simulink model "ddc_model"  (R2023b)
settings: Solver=VariableStepDiscrete  StartTime=0.0  StopTime=DDC_LINEUP_param.endTime  RelTol=1e-3  EnableMultiTasking=on
PreLoadFcn:
  | % Run the setup script when the model is opened
  | setup_ddc_model;
InitFcn:
  | % Run the setup script again just before the
  | % model is run, so that any updates made
  | % after opening are applied.
  | 
  | setup_ddc_model;
StopFcn:
  | ddc_output_analysis;
values from neighbouring files (symbols this model uses):
  DDC_CM_multiplication_factor = 1    [setup_ddc_model.m]
  DDC_CM_NCO1_phase = [0 0 0 0]*2^DDC_LINEUP_param.Complex_NCO1.accum_bit_width    [setup_ddc_model.m]
  DDC_CM_NCO_sync = [0 0 0 0]    [setup_ddc_model.m]
  DDC_CM_number_of_bits_to_shift_left = 0    [setup_ddc_model.m]
undefined symbols (not defined in the file or in its folder): AdvDSPBChannelOutDisplay, COMPLEX_MIXER, DDC_LINEUP_param, dpoly, dspba_ChannelInVis, dspba_ChannelOutVis, dspba_internal_get_channel_ports, evalAionMaskParam, latency, lddc, lddc_lib, mixer_lib, primtype, value
libraries: DSPBAPrim x43, DSPBABase x15, simulink x10, DSPBAFilters x6, DSPBAModelBus x3, DSPBAWaveformSynth x2
(part 1 of 2)
Description:
  | DSP Builder Advanced Template for Template Design implementing ModelIP designs
settings Model: Creator=mjervis  LastModifiedBy=5g
settings SolverCC: AlgebraicLoopSolver=TrustRegion
settings DataIOCC: LimitDataPoints=on  SaveFormat=Array  SignalLoggingSaveFormat=ModelDataLogs  ReturnWorkspaceOutputs=off
settings OptimizationCC: ExpressionDepthLimit=2147483647  LifeSpan=inf
settings DebuggingCC: UnderspecifiedInitializationDetection=Classic  MergeDetectMultiDrivingBlocksExec=none  SolverPrmCheckMsg=warning  InheritedTsInSrcMsg=none  IntegerOverflowMsg=none  FcnCallInpInsideContextMsg=warning  UnconnectedInputMsg=warning  UnconnectedOutputMsg=warning  UnconnectedLineMsg=warning  StateNameClashWarn=warning  SFUnexpectedBacktrackingDiag=warning  SFNoUnconditionalDefaultTransitionDiag=warning  SFExecutionAtInitializationDiag=none  IntegerSaturationMsg=none  ArithmeticOperatorsInVariantConditions=warning
settings HardwareCC: ProdBitPerPointer=32  ProdBitPerSizeT=32  ProdBitPerPtrDiffT=32  ProdLargestAtomicFloat=None  ProdIntDivRoundTo=Undefined  ProdEndianess=Unspecified  ProdWordSize=32  ProdHWDeviceType=32-bit Generic
settings ModelReferenceCC: EnableRefExpFcnMdlSchedulingChecks=on  PropagateSignalLabelsOutOfModel=off
settings SFSimCC: SimUseLocalCustomCode=off  CustomCodeUndefinedFunction=UseInterfaceOnly
settings RTWCC: RTWUseLocalCustomCode=off  DLArmComputeVersion=19.05
settings CodeAppCC: StateflowObjectComments=on
settings GRTTargetCC: TargetLangStandard=C89/C90 (ANSI)  CombineOutputUpdateFcns=off  GRTInterface=on
settings ConfigComp: CovMetricSettings=dw  CovSaveCumulativeToWorkspaceVar=on  CovSaveSingleToWorkspaceVar=on  CovExternalEMLEnable=off

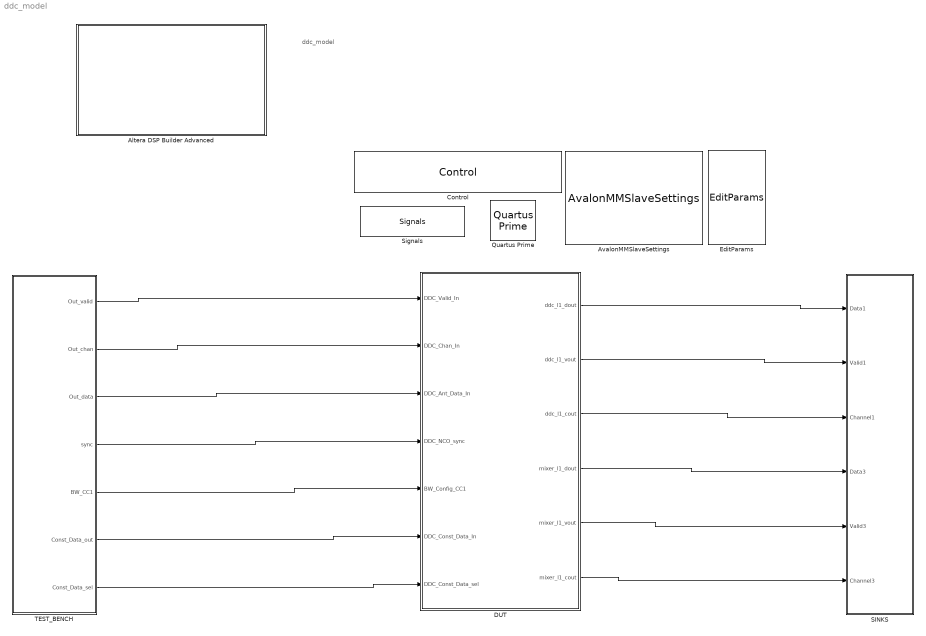
== system ddc_model ==
  note: ddc_model
  Altera DSP Builder Advanced : Subsystem  mask(DSP Builder Advanced Blockset Ignored Block){}
      settings: OpenFcn=web('http://www.altera.com', '-new');
      mask Display: image(imread('intellogo.tif'));
  AvalonMMSlaveSettings : DSPBABase/AvalonMMSlaveSettings
  Control : DSPBABase/Control  generate=on  language=VHDL  destination=./rtl  destination_gui=./rtl  make_full_path=off  path_is_relative=on  autotestbench=on  signaldepth=2  coveragetestbench=off  logs=off  spacewidth=2  spacenum=1  addrwidth=14  datawidth=32  dataendian=Big Endian  hierarchicalnames=off  ramThresholdBits=-1  distRamThresholdBits=-1  mlabThresholdBits=-1  hardMultiplierThresholdLuts=-1  version=20090407  errorOnChanMismatch=1  errorOnGPIOMismatch=0  importModelsimResults=0  cycleAccurate=off  reinterpretCastMult=off  paramFile=ddc_model_params.xml
  DUT : Subsystem
  EditParams : DSPBABase/EditParams  version=20090407
  Quartus Prime : DSPBABase/Quartus Prime  version=20090407
  SINKS : Subsystem
  Signals : DSPBABase/Signals  clk=clk  freq=240  margin=0  rst=areset  rstactive=High  bus=bus  enbusclock=off  busfreq=491.52  bussync=off  version=20090407
  TEST_BENCH : Subsystem
  wires:
  DUT/1(ddc_l1_dout) -> SINKS/1(Data1)
  DUT/2(ddc_l1_vout) -> SINKS/2(Valid1)
  DUT/3("ddc_l1_cout ") -> SINKS/3(Channel1)
  TEST_BENCH/1(Out_valid) -> DUT/1(DDC_Valid_In)
  TEST_BENCH/2(Out_chan) -> DUT/2(DDC_Chan_In)
  TEST_BENCH/3(Out_data) -> DUT/3(DDC_Ant_Data_In)
  TEST_BENCH/4(sync) -> DUT/4(DDC_NCO_sync)
  DUT/4(mixer_l1_dout) -> SINKS/4(Data3)
  DUT/5(mixer_l1_vout) -> SINKS/5(Valid3)
  DUT/6(mixer_l1_cout) -> SINKS/6(Channel3)
  TEST_BENCH/5(BW_CC1) -> DUT/5(BW_Config_CC1)
  TEST_BENCH/6(Const_Data_out) -> DUT/6(DDC_Const_Data_In)
  TEST_BENCH/7(Const_Data_sel) -> DUT/7(DDC_Const_Data_sel)

== system ddc_model/Altera DSP Builder Advanced ==

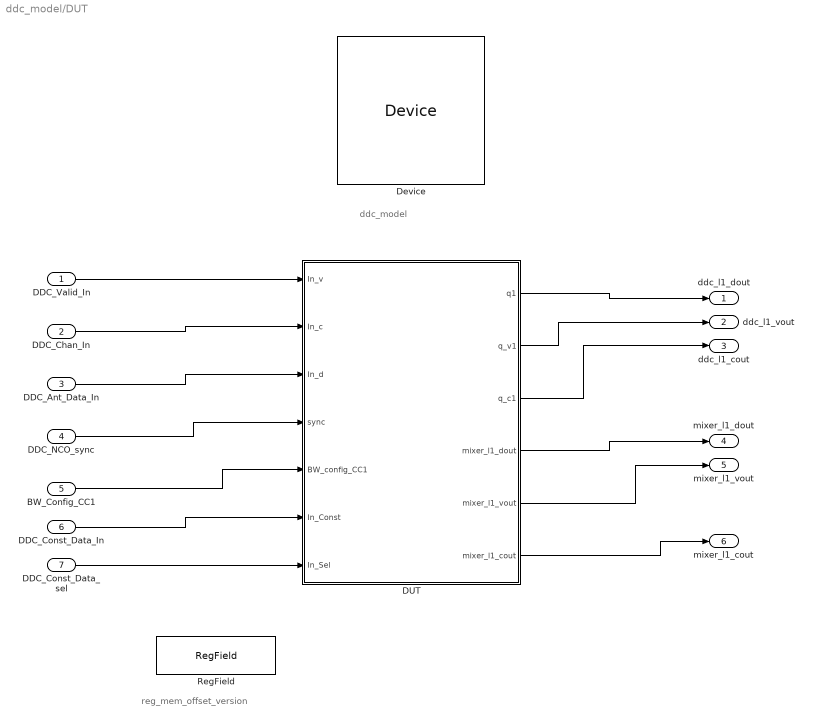
== system ddc_model/DUT ==
  note: ddc_model
  note: reg_mem_offset_version
  DDC_Valid_In : Inport
  DDC_Chan_In : Inport  Port=2
  DDC_Ant_Data_In : Inport  Port=3
  DDC_NCO_sync : Inport  Port=4
  BW_Config_CC1 : Inport  Port=5
  DDC_Const_Data_In : Inport  Port=6
  DDC_Const_Data_sel : Inport  Port=7
  DUT : Subsystem
  Device : DSPBABase/Device  family=Arria 10  deviceMember=Stratix V GX  stratix4device=Stratix IV GX  hardcopy4device=HardCopy IV E  stratix5device=Stratix V GX  device=10AS066N2F40I1SGES  speed=1  stratixSpeed=-5  stratix2Speed=-3  stratix3Speed=-3  stratix4gxSpeed=-2  stratix4gtSpeed=-1  cyclone2Speed=-6  cyclone3Speed=-7  arria2Speed=-4  cyclone4eSpeed=-8  stratix5Speed=-3  arria5Speed=-4  arriaSpeed=-6  cyclone3lsSpeed=-7  cyclone5Speed=-6  arria2gzSpeed=-3  nightFurySpeed=-2  ecp2Speed=-7  hardcopycompat=off  version=20140217  max10flashmode=off  max10nomeminit=off
  RegField : DSPBAModelBus/RegField  reg_name=DDC_LINEUP_param.reg_version.mem_offset  reg_rwmode=Read/Write  reg_msb=31  reg_lsb=0  reg_mode=Specify via dialog  reg_type=ufix(32)  reg_scale=2^0  reg_init=DDC_LINEUP_param.reg_version.Version_reg_val  reg_desc=Version_Output  reg_modal=off  reg_desc0=0  reg_desc1=0  reg_desc2=0  reg_desc3=0  reg_desc4=0  reg_desc5=0  reg_desc6=0  reg_desc7=0  reg_addr=808  SampleTime=-1  version=20090407
  ddc_l1_dout : Outport
  ddc_l1_vout : Outport  Port=2
  "ddc_l1_cout " : Outport  Port=3
  mixer_l1_dout : Outport  Port=4
  mixer_l1_vout : Outport  Port=5
  mixer_l1_cout : Outport  Port=6
  wires:
  DDC_Valid_In/1 -> DUT/1(In_v)
  DDC_Chan_In/1 -> DUT/2(In_c)
  DDC_Ant_Data_In/1 -> DUT/3(In_d)
  DUT/2(q_v1) -> ddc_l1_vout/1
  DUT/1(q1) -> ddc_l1_dout/1
  DUT/3(q_c1) -> "ddc_l1_cout "/1
  DUT/4(mixer_l1_dout) -> mixer_l1_dout/1
  DUT/5(mixer_l1_vout) -> mixer_l1_vout/1
  DUT/6(mixer_l1_cout) -> mixer_l1_cout/1
  DDC_NCO_sync/1 -> DUT/4(sync)
  BW_Config_CC1/1 -> DUT/5(BW_config_CC1)
  DDC_Const_Data_In/1 -> DUT/6(In_Const)
  DDC_Const_Data_sel/1 -> DUT/7(In_Sel)

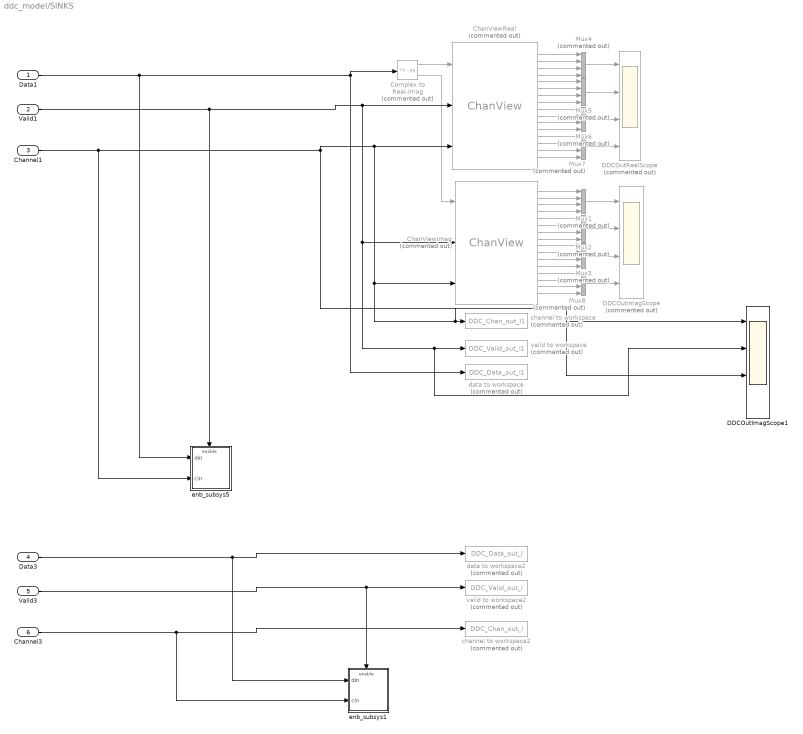
== system ddc_model/SINKS ==
  Data1 : Inport
  Valid1 : Inport  Port=2
  Channel1 : Inport  Port=3
  Data3 : Inport  Port=4
  Valid3 : Inport  Port=5
  Channel3 : Inport  Port=6
  ChanViewImag : DSPBABase/ChanView  Commented=on  nchans=16  chan_vector=[0:15]  outsvalid=off  latency=1  version=20090407
  ChanViewReal : DSPBABase/ChanView  Commented=on  nchans=16  chan_vector=[0:15]  outsvalid=off  latency=1  version=20090407
  Complex to Real-Imag : ComplexToRealImag  Commented=on
  DDCOutImagScope : Scope  Commented=on  NumInputPorts=4
  DDCOutImagScope1 : Scope  NumInputPorts=4
  DDCOutRealScope : Scope  Commented=on  NumInputPorts=4
  Mux{1..8} (8 alike) : Mux  Commented=on
  channel to workspace : ToWorkspace  Commented=on  VariableName=DDC_Chan_out_l1  SaveFormat=Timeseries  SampleTime=-1
  channel to workspace2 : ToWorkspace  Commented=on  VariableName=DDC_Chan_out_l  SaveFormat=Timeseries  SampleTime=-1
  data to workspace : ToWorkspace  Commented=on  VariableName=DDC_Data_out_l1  SaveFormat=Timeseries  SampleTime=-1
  data to workspace2 : ToWorkspace  Commented=on  VariableName=DDC_Data_out_l  SaveFormat=Timeseries  SampleTime=-1
  enb_subsys1 : Subsystem
  enb_subsys5 : Subsystem
  valid to workspace : ToWorkspace  Commented=on  VariableName=DDC_Valid_out_l1  SaveFormat=Timeseries  SampleTime=-1
  valid to workspace2 : ToWorkspace  Commented=on  VariableName=DDC_Valid_out_l  SaveFormat=Timeseries  SampleTime=-1
  wires:
  Mux7/1 -> DDCOutRealScope/4
  ChanViewReal/14 -> Mux7/2
  ChanViewReal/15 -> Mux7/3
  ChanViewReal/16 -> Mux7/4
  ChanViewReal/13 -> Mux7/1
  Mux6/1 -> DDCOutRealScope/3
  ChanViewReal/11 -> Mux6/3
  ChanViewReal/12 -> Mux6/4
  ChanViewReal/9 -> Mux6/1
  ChanViewReal/10 -> Mux6/2
  Mux5/1 -> DDCOutRealScope/2
  ChanViewReal/6 -> Mux5/2
  ChanViewReal/7 -> Mux5/3
  ChanViewReal/5 -> Mux5/1
  ChanViewReal/8 -> Mux5/4
  Mux4/1 -> DDCOutRealScope/1
  ChanViewReal/3 -> Mux4/3
  ChanViewReal/4 -> Mux4/4
  ChanViewReal/2 -> Mux4/2
  ChanViewReal/1 -> Mux4/1
  Complex to Real-Imag/2 -> ChanViewImag/1
  Complex to Real-Imag/1 -> ChanViewReal/1
  Data1/1 -> enb_subsys5/1(din), Complex to Real-Imag/1, data to workspace/1
  Channel1/1 -> enb_subsys5/2(cin), DDCOutImagScope1/1, channel to workspace/1, ChanViewImag/3, ChanViewReal/3, DDCOutImagScope1/3
  Valid1/1 -> ChanViewReal/2, DDCOutImagScope1/2, valid to workspace/1, ChanViewImag/2, enb_subsys5/Enable
  Mux8/1 -> DDCOutImagScope/4
  ChanViewImag/14 -> Mux8/2
  ChanViewImag/15 -> Mux8/3
  ChanViewImag/16 -> Mux8/4
  ChanViewImag/13 -> Mux8/1
  Mux3/1 -> DDCOutImagScope/3
  ChanViewImag/11 -> Mux3/3
  ChanViewImag/12 -> Mux3/4
  ChanViewImag/9 -> Mux3/1
  ChanViewImag/10 -> Mux3/2
  Mux2/1 -> DDCOutImagScope/2
  ChanViewImag/6 -> Mux2/2
  ChanViewImag/7 -> Mux2/3
  ChanViewImag/5 -> Mux2/1
  ChanViewImag/8 -> Mux2/4
  Mux1/1 -> DDCOutImagScope/1
  ChanViewImag/3 -> Mux1/3
  ChanViewImag/4 -> Mux1/4
  ChanViewImag/2 -> Mux1/2
  ChanViewImag/1 -> Mux1/1
  Data3/1 -> enb_subsys1/1(din), data to workspace2/1
  Channel3/1 -> enb_subsys1/2(cin), channel to workspace2/1
  Valid3/1 -> enb_subsys1/Enable, valid to workspace2/1

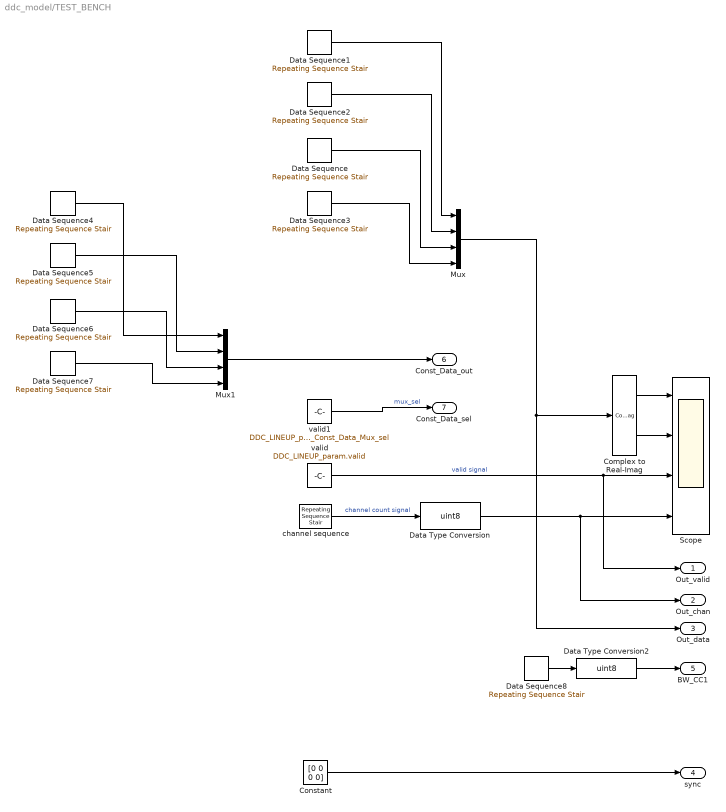
== system ddc_model/TEST_BENCH ==
  Complex to Real-Imag : ComplexToRealImag
  Constant : Constant  Value=[0 0 0 0]  OutDataTypeStr=boolean
  Data Sequence : simulink/Sources/Repeating Sequence Stair  OutValues=DDC_LINEUP_param.DDC_Ant_Data_in_3  tsamp=DDC_LINEUP_param.SampleTime  OutMin=[]  OutMax=[]  OutDataTypeStr=fixdt(1,DDC_LINEUP_param.input_word_length,DDC_LINEUP_param.input_fraction_length)  OutputDataTypeScalingMode=Specify via dialog  OutDataType=fixdt(1,DDC_LINEUP_param.input_word_length,DDC_LINEUP_param.input_fraction_length)  ConRadixGroup=Best Precision: Vector-wise  OutScaling=[]
  Data Sequence1 : simulink/Sources/Repeating Sequence Stair  OutValues=DDC_LINEUP_param.DDC_Ant_Data_in_1  tsamp=DDC_LINEUP_param.SampleTime  OutMin=[]  OutMax=[]  OutDataTypeStr=fixdt(1,DDC_LINEUP_param.input_word_length,DDC_LINEUP_param.input_fraction_length)  OutputDataTypeScalingMode=Specify via dialog  OutDataType=fixdt(1,DDC_LINEUP_param.input_word_length,DDC_LINEUP_param.input_fraction_length)  ConRadixGroup=Best Precision: Vector-wise  OutScaling=[]
  Data Sequence2 : simulink/Sources/Repeating Sequence Stair  OutValues=DDC_LINEUP_param.DDC_Ant_Data_in_2  tsamp=DDC_LINEUP_param.SampleTime  OutMin=[]  OutMax=[]  OutDataTypeStr=fixdt(1,DDC_LINEUP_param.input_word_length,DDC_LINEUP_param.input_fraction_length)  OutputDataTypeScalingMode=Specify via dialog  OutDataType=fixdt(1,DDC_LINEUP_param.input_word_length,DDC_LINEUP_param.input_fraction_length)  ConRadixGroup=Best Precision: Vector-wise  OutScaling=[]
  Data Sequence3 : simulink/Sources/Repeating Sequence Stair  OutValues=DDC_LINEUP_param.DDC_Ant_Data_in_4  tsamp=DDC_LINEUP_param.SampleTime  OutMin=[]  OutMax=[]  OutDataTypeStr=fixdt(1,DDC_LINEUP_param.input_word_length,DDC_LINEUP_param.input_fraction_length)  OutputDataTypeScalingMode=Specify via dialog  OutDataType=fixdt(1,DDC_LINEUP_param.input_word_length,DDC_LINEUP_param.input_fraction_length)  ConRadixGroup=Best Precision: Vector-wise  OutScaling=[]
  Data Sequence4 : simulink/Sources/Repeating Sequence Stair  OutValues=DDC_LINEUP_param.DDC_Const_Data_in_1  tsamp=DDC_LINEUP_param.SampleTime  OutMin=[]  OutMax=[]  OutDataTypeStr=fixdt(1,DDC_LINEUP_param.input_word_length,DDC_LINEUP_param.input_fraction_length)  OutputDataTypeScalingMode=Specify via dialog  OutDataType=fixdt(1,DDC_LINEUP_param.input_word_length,DDC_LINEUP_param.input_fraction_length)  ConRadixGroup=Best Precision: Vector-wise  OutScaling=[]
  Data Sequence5 : simulink/Sources/Repeating Sequence Stair  OutValues=DDC_LINEUP_param.DDC_Const_Data_in_2  tsamp=DDC_LINEUP_param.SampleTime  OutMin=[]  OutMax=[]  OutDataTypeStr=fixdt(1,DDC_LINEUP_param.input_word_length,DDC_LINEUP_param.input_fraction_length)  OutputDataTypeScalingMode=Specify via dialog  OutDataType=fixdt(1,DDC_LINEUP_param.input_word_length,DDC_LINEUP_param.input_fraction_length)  ConRadixGroup=Best Precision: Vector-wise  OutScaling=[]
  Data Sequence6 : simulink/Sources/Repeating Sequence Stair  OutValues=DDC_LINEUP_param.DDC_Const_Data_in_3  tsamp=DDC_LINEUP_param.SampleTime  OutMin=[]  OutMax=[]  OutDataTypeStr=fixdt(1,DDC_LINEUP_param.input_word_length,DDC_LINEUP_param.input_fraction_length)  OutputDataTypeScalingMode=Specify via dialog  OutDataType=fixdt(1,DDC_LINEUP_param.input_word_length,DDC_LINEUP_param.input_fraction_length)  ConRadixGroup=Best Precision: Vector-wise  OutScaling=[]
  Data Sequence7 : simulink/Sources/Repeating Sequence Stair  OutValues=DDC_LINEUP_param.DDC_Const_Data_in_4  tsamp=DDC_LINEUP_param.SampleTime  OutMin=[]  OutMax=[]  OutDataTypeStr=fixdt(1,DDC_LINEUP_param.input_word_length,DDC_LINEUP_param.input_fraction_length)  OutputDataTypeScalingMode=Specify via dialog  OutDataType=fixdt(1,DDC_LINEUP_param.input_word_length,DDC_LINEUP_param.input_fraction_length)  ConRadixGroup=Best Precision: Vector-wise  OutScaling=[]
  Data Sequence8 : simulink/Sources/Repeating Sequence Stair  OutValues=BW_Config_CC1  tsamp=DDC_LINEUP_param.SampleTime  OutMin=[]  OutMax=[]  OutDataTypeStr=uint(8)  OutputDataTypeScalingMode=Specify via dialog  OutDataType=uint(8)  ConRadixGroup=Best Precision: Vector-wise  OutScaling=[]
  Data Type Conversion : DataTypeConversion  OutDataTypeStr=uint8  SaturateOnIntegerOverflow=off  RndMeth=Floor
  Data Type Conversion2 : DataTypeConversion  OutDataTypeStr=uint8  SaturateOnIntegerOverflow=off  RndMeth=Floor
  Mux : Mux
  Mux1 : Mux
  Scope : Scope  NumInputPorts=4
  channel sequence : simulink/Sources/Repeating Sequence Stair  OutValues=DDC_LINEUP_param.channel  tsamp=DDC_LINEUP_param.SampleTime  OutMin=[]  OutMax=[]  OutDataTypeStr=uint8  OutputDataTypeScalingMode=uint8  OutDataType=fixdt(1,16)  ConRadixGroup=Best Precision: Vector-wise  OutScaling=[]
  valid : Constant  Value=DDC_LINEUP_param.valid  OutDataTypeStr=boolean  SampleTime=DDC_LINEUP_param.SampleTime
  valid1 : Constant  Value=DDC_LINEUP_param.DDC_Const_Data_Mux_sel  OutDataTypeStr=boolean  SampleTime=DDC_LINEUP_param.SampleTime
  Out_valid : Outport
  Out_chan : Outport  Port=2
  Out_data : Outport  Port=3
  sync : Outport  Port=4
  BW_CC1 : Outport  Port=5
  Const_Data_out : Outport  Port=6
  Const_Data_sel : Outport  Port=7
  wires:
  Complex to Real-Imag/1 -> Scope/1
  valid/1 -> Scope/3, Out_valid/1  "valid signal"
  channel sequence/1 -> Data Type Conversion/1  "channel count signal"
  Data Type Conversion/1 -> Scope/4, Out_chan/1
  Complex to Real-Imag/2 -> Scope/2
  Mux/1 -> Complex to Real-Imag/1, Out_data/1
  Data Sequence3/1 -> Mux/4
  Data Sequence/1 -> Mux/3
  Data Sequence2/1 -> Mux/2
  Data Sequence1/1 -> Mux/1
  Constant/1 -> sync/1
  Data Sequence8/1 -> Data Type Conversion2/1
  Data Type Conversion2/1 -> BW_CC1/1
  Data Sequence5/1 -> Mux1/2
  Data Sequence7/1 -> Mux1/4
  Data Sequence6/1 -> Mux1/3
  Mux1/1 -> Const_Data_out/1
  Data Sequence4/1 -> Mux1/1
  valid1/1 -> Const_Data_sel/1  "mux_sel"

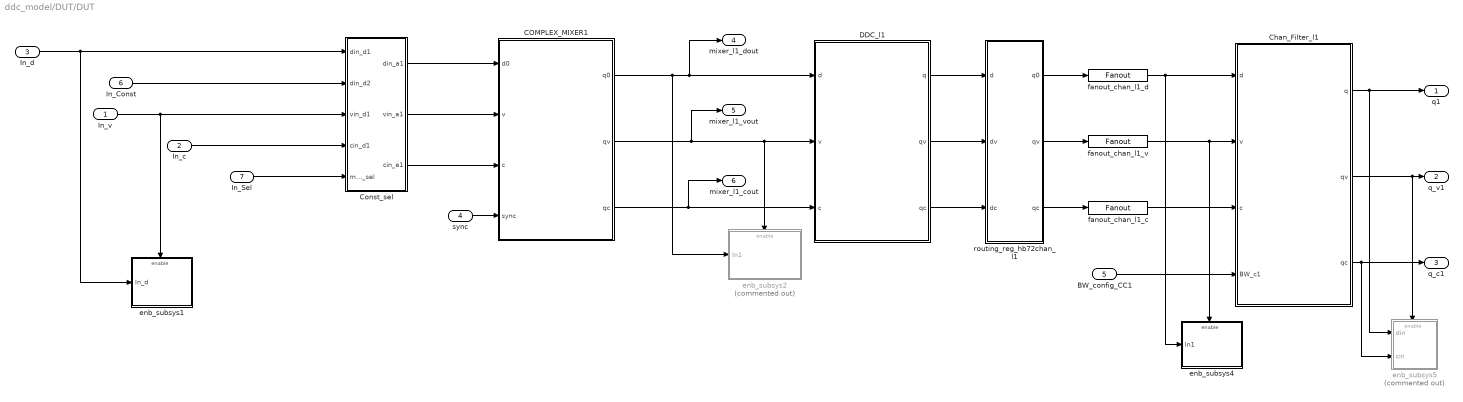
== system ddc_model/DUT/DUT ==
  In_v : Inport
  In_c : Inport  Port=2
  In_d : Inport  Port=3
  sync : Inport  Port=4
  BW_config_CC1 : Inport  Port=5
  In_Const : Inport  Port=6
  In_Sel : Inport  Port=7
  COMPLEX_MIXER1 : Subsystem  AncestorBlock=mixer_lib/COMPLEX_MIXER  mask{CM_clock_margin=DDC_LINEUP_param.ClockMargin, CM_NCO_sample_rate=DDC_LINEUP_param.Complex_NCO1.sample_rate, CM_NCO_accumulator_bit_width=DDC_LINEUP_param.Complex_NCO1.accum_bit_width, CM_NCO_frequency_word=DDC_LINEUP_param.Complex_NCO1.ph_incrandInv, CM_NCO_base_addr=DDC_LINEUP_param.Complex_NCO1.base_addr, CM_NCO_data_type=DDC_LINEUP_param.Complex_NCO1.data_type, CM_NCO_scaling_value=DDC_LINEUP_param.Complex_NCO1.scaling_value, CM_sample_rate=DDC_LINEUP_param.CM.SampleRate, CM_complex_channels=DDC_LINEUP_param.CM.num_complex_chans, CM_complex_freq=DDC_LINEUP_param.CM.num_complex_freqs, CM_output_word_length=DDC_LINEUP_param.output_word_length, CM_output_fraction_length=DDC_LINEUP_param.output_fraction_length, CM_scale_multiplication_factor=DDC_CM_multiplication_factor, CM_scale_left_shift_factor=DDC_CM_number_of_bits_to_shift_left, CM_NCO_phase=DDC_CM_NCO1_phase, CM_NCO_sync=DDC_CM_NCO_sync}
      mask prompts: CM_clock_margin "Clock margin"; CM_NCO_sample_rate "NCO sample rate"; CM_NCO_accumulator_bit_width "NCO accumulator bit width"; CM_NCO_frequency_word "NCO Frequency word"; CM_NCO_base_addr "NCO base address"; CM_NCO_data_type "NCO data type"; CM_NCO_scaling_value "NCO scaling value"; CM_sample_rate "Sample Rate"; CM_complex_channels "Number of complex channels"; CM_complex_freq "Number of complex frequencies"; CM_output_word_length "Output word length"; CM_output_fraction_length "Output fraction length"; CM_scale_multiplication_factor "Scale multiplication factor"; CM_scale_left_shift_factor "Scale left-shift factor"; CM_NCO_phase "NCO phase"; CM_NCO_sync "NCO sync"
      mask Display:
      | disp('COMPLEX\nMIXER');
      | port_label('input',1,'d0');
      | port_label('input',2,'v');
      | port_label('input',3,'c');
      | port_label('input',4,'sync');
      | 
      | 
      | port_label('output',1,'q0');
      | port_label('output',2,'qv');
      | port_label('output',3,'qc');
  Chan_Filter_l1 : Subsystem  AncestorBlock=lddc_lib/lddc  mask{CH_filter_SampleRate=DDC_LINEUP_param.chan_filter.SampleRate, CH_filter_base_addr_l1_re=DDC_LINEUP_param.chan_filter.chan_filt_base_addr_l1_re, CH_filter_base_addr_l1_im=DDC_LINEUP_param.chan_filter.chan_filt_base_addr_l1_im, CH_filter_ChanCount=DDC_LINEUP_param.chan_filter.ChanCount, CH_filter_coeffs=DDC_LINEUP_param.chan_filter.coeffs, output_word_length=DDC_LINEUP_param.output_word_length, output_fraction_length=DDC_LINEUP_param.output_fraction_length, Pipeline_stages=2, Clock_Margin=DDC_LINEUP_param.ClockMargin}
      mask Display:
      | disp('DDC');
      | port_label('input',1,'d');
      | port_label('input',2,'v');
      | port_label('input',3,'c');
      | 
      | 
      | port_label('output',1,'q1');
      | port_label('output',2,'q_v');
      | port_label('output',3,'q_c');
  Const_sel : Subsystem
  "DDC_l1 " : Subsystem
  enb_subsys1 : Subsystem
  enb_subsys2 : Subsystem  Commented=on
  enb_subsys4 : Subsystem
  enb_subsys5 : Subsystem  Commented=on
  fanout_chan_l1_c : DSPBAPrim/Fanout  primtype=fanout  nInputs=1  nOutputs=evalAionMaskParam(gcb,'value',1)  omode=Inherit via internal rule  otype=sfix(16)  scale=2^-15  rndmethod=Unbiased  factor=1  satmethod=Symmetric  shift_vec=[0 1 2 -1]  value=1  inPortNames=[' '; ' ';]  outPortNames=[' ']  dspbaimage=dspba_prim_tall.svg  text=fprintf('fanout')  style=Optimised  visibilities=2^10+2^18  version=20211007  uninit=off
  fanout_chan_l1_d : DSPBAPrim/Fanout  primtype=fanout  nInputs=1  nOutputs=evalAionMaskParam(gcb,'value',1)  omode=Inherit via internal rule  otype=sfix(16)  scale=2^-15  rndmethod=Unbiased  factor=1  satmethod=Symmetric  shift_vec=[0 1 2 -1]  value=1  inPortNames=[' '; ' ';]  outPortNames=[' ']  dspbaimage=dspba_prim_tall.svg  text=fprintf('fanout')  style=Optimised  visibilities=2^10+2^18  version=20211007  uninit=off
  fanout_chan_l1_v : DSPBAPrim/Fanout  primtype=fanout  nInputs=1  nOutputs=evalAionMaskParam(gcb,'value',1)  omode=Inherit via internal rule  otype=sfix(16)  scale=2^-15  rndmethod=Unbiased  factor=1  satmethod=Symmetric  shift_vec=[0 1 2 -1]  value=1  inPortNames=[' '; ' ';]  outPortNames=[' ']  dspbaimage=dspba_prim_tall.svg  text=fprintf('fanout')  style=Optimised  visibilities=2^10+2^18  version=20211007  uninit=off
  routing_reg_hb72chan_l1 : Subsystem
  q1 : Outport
  q_v1 : Outport  Port=2
  q_c1 : Outport  Port=3
  mixer_l1_dout : Outport  Port=4
  mixer_l1_vout : Outport  Port=5
  mixer_l1_cout : Outport  Port=6
  wires:
  COMPLEX_MIXER1/1(q0) -> enb_subsys2/1(In1), mixer_l1_dout/1, "DDC_l1 "/1(d)
  COMPLEX_MIXER1/3(qc) -> mixer_l1_cout/1, "DDC_l1 "/3(c)
  Chan_Filter_l1/1(q) -> enb_subsys5/1(din), q1/1
  Chan_Filter_l1/2(qv) -> enb_subsys5/Enable, q_v1/1
  Chan_Filter_l1/3(qc) -> enb_subsys5/2(cin), q_c1/1
  COMPLEX_MIXER1/2(qv) -> mixer_l1_vout/1, enb_subsys2/Enable, "DDC_l1 "/2(v)
  sync/1 -> COMPLEX_MIXER1/4(sync)
  In_c/1 -> Const_sel/4(cin_d1)
  In_v/1 -> enb_subsys1/Enable, Const_sel/3(vin_d1)
  In_d/1 -> enb_subsys1/1(In_d), Const_sel/1(din_d1)
  "DDC_l1 "/1(q) -> routing_reg_hb72chan_l1/1(d)
  routing_reg_hb72chan_l1/3(qc) -> fanout_chan_l1_c/1
  routing_reg_hb72chan_l1/1(q0) -> fanout_chan_l1_d/1
  routing_reg_hb72chan_l1/2(qv) -> fanout_chan_l1_v/1
  "DDC_l1 "/3(qc) -> routing_reg_hb72chan_l1/3(dc)
  "DDC_l1 "/2(qv) -> routing_reg_hb72chan_l1/2(dv)
  fanout_chan_l1_d/1 -> enb_subsys4/1(In1), Chan_Filter_l1/1(d)
  fanout_chan_l1_v/1 -> enb_subsys4/Enable, Chan_Filter_l1/2(v)
  fanout_chan_l1_c/1 -> Chan_Filter_l1/3(c)
  BW_config_CC1/1 -> Chan_Filter_l1/4(BW_c1)
  In_Sel/1 -> Const_sel/5(mux_sel)
  In_Const/1 -> Const_sel/2(din_d2)
  Const_sel/3(cin_a1) -> COMPLEX_MIXER1/3(c)
  Const_sel/2(vin_a1) -> COMPLEX_MIXER1/2(v)
  Const_sel/1(din_a1) -> COMPLEX_MIXER1/1(d0)

== system ddc_model/SINKS/enb_subsys1 ==
  din : Inport
  cin : Inport  Port=2
  Enable : EnablePort
  To Workspace : ToWorkspace  VariableName=mixer_out1  SampleTime=-1
      settings: Save2DSignal=2-D array (concatenate along first dimension)
  To Workspace1 : ToWorkspace  VariableName=mixer_out1_cout  SampleTime=-1
      settings: Save2DSignal=2-D array (concatenate along first dimension)
  wires:
  cin/1 -> To Workspace1/1
  din/1 -> To Workspace/1

== system ddc_model/SINKS/enb_subsys5 ==
  din : Inport
  cin : Inport  Port=2
  Enable : EnablePort
  To Workspace : ToWorkspace  VariableName=chFiltOut  SampleTime=-1
      settings: Save2DSignal=2-D array (concatenate along first dimension)
  To Workspace1 : ToWorkspace  VariableName=chFiltOut_cout  SampleTime=-1
      settings: Save2DSignal=2-D array (concatenate along first dimension)
  wires:
  din/1 -> To Workspace/1
  cin/1 -> To Workspace1/1

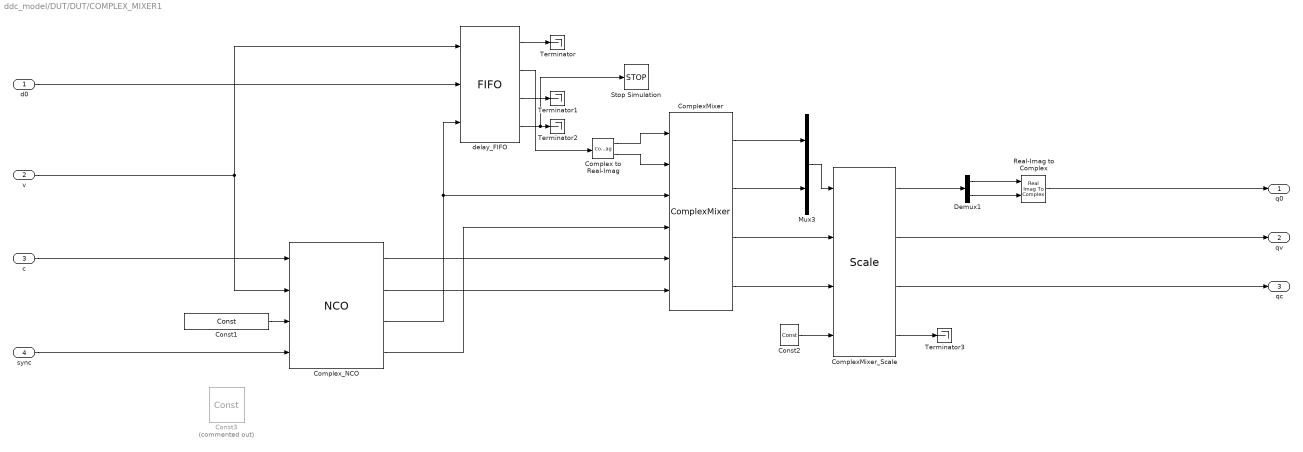
== system ddc_model/DUT/DUT/COMPLEX_MIXER1 ==
  d0 : Inport
  v : Inport  Port=2
  c : Inport  Port=3
  sync : Inport  Port=4
  Complex to Real-Imag : ComplexToRealImag
  ComplexMixer : DSPBAWaveformSynth/ComplexMixer  nInputRate=CM_sample_rate  nchan=CM_complex_channels  nfreq=CM_complex_freq  latency=8  simulationMode=Use Global Value  version=20090407
  ComplexMixer_Scale : DSPBABase/Scale  otype=sfix(CM_output_word_length)  scale=2^-CM_output_fraction_length  rndmethod=Biased  factor=CM_scale_multiplication_factor  satmethod=None  shift_vec=CM_scale_left_shift_factor  latency=2  simulationMode=Use Global Value  version=20130807
  Complex_NCO : DSPBAWaveformSynth/NCO  outputRate=CM_NCO_sample_rate  otype=sfix(CM_NCO_data_type)  scale=2^-CM_NCO_scaling_value  accumBitWidth=CM_NCO_accumulator_bit_width  phaseIncrAndInv=CM_NCO_frequency_word  phaseIncrAndInvMap=CM_NCO_base_addr  rwmode=Read/Write  exposebus=off  version=20090407  SampleTime=-1  expSFDR=96.32  accumPrecision=+/- 0.05722  phaseIncrInMHz="[1033.04       50  1033.04       50]"  outWidth=4  tableSize=8  latency=17
      settings: AttributesFormatString=%<latency>
  Const1 : DSPBAPrim/Const  primtype=const  nInputs=0  nOutputs=1  omode=Specify via dialog  otype=ufix(32)  scale=2^-0  rndmethod=Unbiased  factor=1  satmethod=Symmetric  shift_vec=[0 1 2 -1]  value=CM_NCO_phase  inPortNames=['+'; '+';]  outPortNames=[' ']  dspbaimage=dspba_prim.svg  text=fprintf('%s', num2str(value));  style=Optimised  visibilities=8 + 1024  floatPrecision=float32_m23  warnSaturation=on  version=20211007  SampleTime=inf
  Const2 : DSPBAPrim/Const  primtype=const  nInputs=0  nOutputs=1  omode=Specify via dialog  otype=ufix(1)  scale=1  rndmethod=Unbiased  factor=1  satmethod=Symmetric  shift_vec=[0 1 2 -1]  value=0  inPortNames=['+'; '+';]  outPortNames=[' ']  dspbaimage=dspba_prim.svg  text=fprintf('%s', num2str(value));  style=Optimised  visibilities=8 + 1024  floatPrecision=float32_m23  warnSaturation=on  version=20211007  SampleTime=inf
  Const3 : DSPBAPrim/Const  Commented=on  primtype=const  nInputs=0  nOutputs=1  omode=boolean  otype=sfix(16)  scale=2^-15  rndmethod=Unbiased  factor=1  satmethod=Symmetric  shift_vec=[0 1 2 -1]  value=[0 0 0 0]  inPortNames=['+'; '+';]  outPortNames=[' ']  dspbaimage=dspba_prim.svg  text=fprintf('%s', num2str(value));  style=Optimised  visibilities=8 + 1024  floatPrecision=float32_m23  warnSaturation=on  version=20211007  SampleTime=inf
  Demux1 : Demux  Outputs=2
  Mux3 : Mux  Inputs=2
  Real-Imag to Complex : RealImagToComplex
  Stop Simulation : Stop
  Terminator{,1..3} (4 alike) : Terminator
  delay_FIFO : DSPBAPrim/FIFO  primtype=fifo  nInputs=3  nOutputs=4  omode=Inherit via internal rule  otype=sfix(16)  scale=2^-15  rndmethod=Unbiased  factor=1  satmethod=Symmetric  shift_vec=[0 1 2 -1]  value=[64 4 63]  inPortNames=['w'; 'd'; 'r'; 'f']  outPortNames=['v'; 'q'; 't'; 'f']  dspbaimage=dspba_prim_tall.svg  text=fprintf('fifo');  style=Optimised  visibilities=263168  version=20211007  user_sclr=off
  q0 : Outport
  qv : Outport  Port=2
  qc : Outport  Port=3
  wires:
  Const1/1 -> Complex_NCO/3
  ComplexMixer/3 -> ComplexMixer_Scale/2
  ComplexMixer/4 -> ComplexMixer_Scale/3
  Mux3/1 -> ComplexMixer_Scale/1
  ComplexMixer/2 -> Mux3/2
  ComplexMixer/1 -> Mux3/1
  Const2/1 -> ComplexMixer_Scale/4
  ComplexMixer_Scale/4 -> Terminator3/1
  Demux1/1 -> Real-Imag to Complex/1
  Demux1/2 -> Real-Imag to Complex/2
  sync/1 -> Complex_NCO/4
  Complex_NCO/3 -> ComplexMixer/3, delay_FIFO/3
  Complex_NCO/4 -> ComplexMixer/4
  ComplexMixer_Scale/3 -> qc/1
  ComplexMixer_Scale/2 -> qv/1
  Real-Imag to Complex/1 -> q0/1
  v/1 -> delay_FIFO/1, Complex_NCO/2
  c/1 -> Complex_NCO/1
  Complex to Real-Imag/1 -> ComplexMixer/1
  Complex to Real-Imag/2 -> ComplexMixer/2
  Complex_NCO/1 -> ComplexMixer/5
  Complex_NCO/2 -> ComplexMixer/6
  ComplexMixer_Scale/1 -> Demux1/1
  delay_FIFO/4 -> Stop Simulation/1, Terminator2/1
  delay_FIFO/3 -> Terminator1/1
  delay_FIFO/1 -> Terminator/1
  delay_FIFO/2 -> Complex to Real-Imag/1
  d0/1 -> delay_FIFO/2

== system ddc_model/DUT/DUT/Chan_Filter_l1 ==
  d : Inport
  v : Inport  Port=2
  c : Inport  Port=3
  BW_c1 : Inport  Port=4
  Chan_Filter : Subsystem
  Filter-Reconfig : Subsystem
  q : Outport
  qv : Outport  Port=2
  qc : Outport  Port=3
  wires:
  Chan_Filter/1(q) -> q/1
  Chan_Filter/2(qv) -> qv/1
  Chan_Filter/3(qc) -> qc/1
  d/1 -> Filter-Reconfig/1(In1)
  v/1 -> Filter-Reconfig/2(v)
  c/1 -> Filter-Reconfig/3(c)
  Filter-Reconfig/2(Out4) -> Chan_Filter/2(v)
  Filter-Reconfig/1(d1) -> Chan_Filter/1(d1)
  Filter-Reconfig/3(Out6) -> Chan_Filter/3(c)
  Filter-Reconfig/4(CoefBankSel) -> Chan_Filter/4(bank)
  BW_c1/1 -> Filter-Reconfig/4(BWconfig_C1)

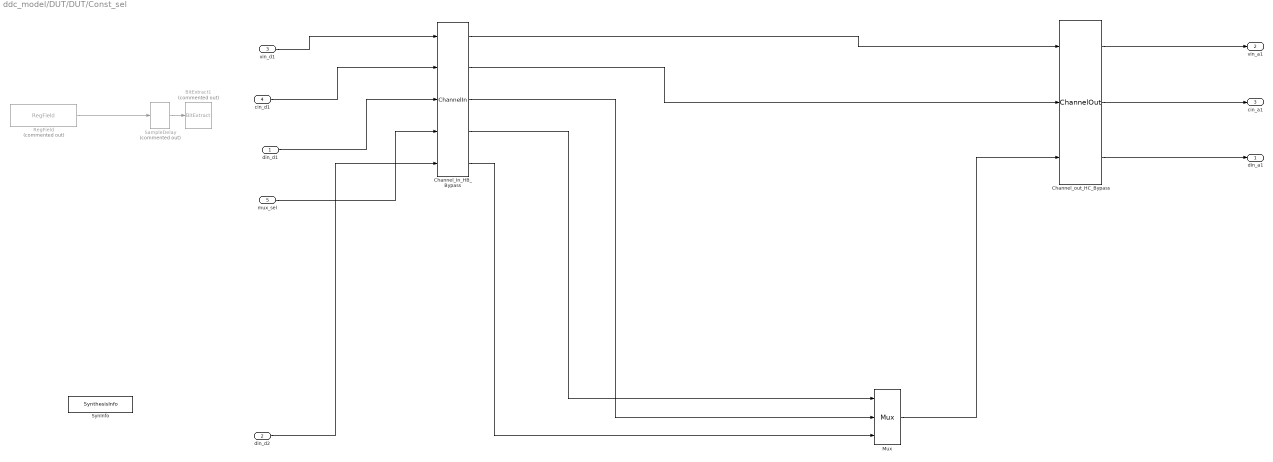
== system ddc_model/DUT/DUT/Const_sel ==
  din_d1 : Inport
  din_d2 : Inport  Port=2
  vin_d1 : Inport  Port=3
  cin_d1 : Inport  Port=4
  mux_sel : Inport  Port=5
  BitExtract1 : DSPBAPrim/BitExtract  Commented=on  primtype=bitextract  nInputs=1  nOutputs=1  omode=boolean  otype=uint(16)  scale=1  rndmethod=Unbiased  factor=1  satmethod=Symmetric  shift_vec=[0 1 2 -1]  value=0  inPortNames=[' '; ' ';]  outPortNames=[' ']  dspbaimage=dspba_prim.svg  text=fprintf('..%d', value);  style=Optimised  visibilities=8+1024  version=20211007
  Channel_In_HB_Bypass : DSPBAPrim/ChannelIn  primtype=channelin  nInputs=dspba_internal_get_channel_ports(gcb)  nOutputs=dspba_internal_get_channel_ports(gcb)  omode=Inherit via internal rule  otype=sfix(16)  scale=2^-15  rndmethod=Unbiased  factor=1  satmethod=Symmetric  shift_vec=[0 1 2 -1]  value=3  inPortNames=['v'; 'c'; '0'; '1'; '2'; '3'; '4'; '5'; '6'; '7'; '8'; '9'; 'A'; 'B'; 'D'; 'E'; 'F'; 'G'; 'H'; 'I'; 'J'; 'K'; 'L'; 'M'; 'N'; 'O'; 'P'; 'Q'; 'R'; 'S'; 'T'; 'U'; 'W'; 'X'; 'Y'; 'Z']  outPortNames=['v'; 'c'; '0'; '1'; '2'; '3'; '4'; '5'; '6'; '7'; '8'; '9'; 'A'; 'B'; 'D'; 'E'; 'F'; 'G'; 'H'; 'I'; 'J'; 'K'; 'L'; 'M'; 'N'; 'O'; 'P'; 'Q'; 'R'; 'S'; 'T'; 'U'; 'W'; 'X'; 'Y'; 'Z']  dspbaimage=dspba_prim_channel_tall.svg  text=fprintf('In');  style=Optimised  dataSignals=3  foldingEnabled=off  channels=1  sampleRate=200  packetBeginPresent=off  packetBeginEnabled=off  visibilities=dspba_ChannelInVis(gcb)  scheduleOrigin=on  version=20211214
  Channel_out_HC_Bypass : DSPBAPrim/ChannelOut  primtype=channelout  nInputs=dspba_internal_get_channel_ports(gcb)  nOutputs=dspba_internal_get_channel_ports(gcb)  omode=Inherit via internal rule  otype=sfix(16)  scale=2^-15  rndmethod=Unbiased  factor=1  satmethod=Symmetric  shift_vec=[0 1 2 -1]  value=1  inPortNames=['v'; 'c'; '0'; '1'; '2'; '3'; '4'; '5'; '6'; '7'; '8'; '9'; 'A'; 'B'; 'D'; 'E'; 'F'; 'G'; 'H'; 'I'; 'J'; 'K'; 'L'; 'M'; 'N'; 'O'; 'P'; 'Q'; 'R'; 'S'; 'T'; 'U'; 'W'; 'X'; 'Y'; 'Z']  outPortNames=['v'; 'c'; '0'; '1'; '2'; '3'; '4'; '5'; '6'; '7'; '8'; '9'; 'A'; 'B'; 'D'; 'E'; 'F'; 'G'; 'H'; 'I'; 'J'; 'K'; 'L'; 'M'; 'N'; 'O'; 'P'; 'Q'; 'R'; 'S'; 'T'; 'U'; 'W'; 'X'; 'Y'; 'Z']  dspbaimage=dspba_prim_channel_tall.svg  text=fprintf('Out%s', AdvDSPBChannelOutDisplay(latency));  style=Optimised  dataSignals=1  foldingEnabled=off  channels=1  sampleRate=200  packetBeginPresent=off  packetBeginEnabled=off  visibilities=dspba_ChannelOutVis(gcb)  latency=0  version=20211214
  Mux : DSPBAPrim/Mux  primtype=mux  nInputs=evalAionMaskParam(gcb,'value',1)+1  nOutputs=1  omode=Inherit via internal rule  otype=sfix(16)  scale=2^-15  rndmethod=Unbiased  factor=1  satmethod=Symmetric  shift_vec=[0 1 2 -1]  value=2  inPortNames=['s '; 'd0'; 'd1'; 'd2'; 'd3'; 'd4'; 'd5'; 'd6'; 'd7'; 'd8'; 'd9';]  outPortNames=[' ']  dspbaimage=dspba_prim_tall.svg  text=fprintf('%s', primtype);  style=Optimised  visibilities=1032  version=20211007
  RegField : DSPBAModelBus/RegField  Commented=on  reg_name=DDC_LINEUP_param.HB_Bypass  reg_rwmode=Read/Write  reg_msb=15  reg_lsb=0  reg_mode=Specify via dialog  reg_type=ufix(16)  reg_scale=2^-0  reg_init=0  reg_desc=Description of what is stored in this field  reg_modal=off  reg_desc0=0  reg_desc1=0  reg_desc2=0  reg_desc3=0  reg_desc4=0  reg_desc5=0  reg_desc6=0  reg_desc7=0  reg_addr=132  SampleTime=-1  version=20090407
  SampleDelay : DSPBAPrim/SampleDelay  Commented=on  primtype=sampdelay  nInputs=1  nOutputs=1  omode=Inherit via internal rule  otype=sfix(16)  scale=2^-15  rndmethod=Unbiased  factor=1  satmethod=Symmetric  shift_vec=[0 1 2 -1]  floatPrecision=float32_m23  value=1  inPortNames=[' '; ' ';]  outPortNames=[' ']  dspbaimage=dspba_prim.svg  text=dpoly(1, eye(1,value+1), 'z')  style=Optimised  visibilities=8 + 1024 + 2^17 + 2^18  flexible=off  slackgroup=0  augmented=0  version=20211007  advOptions=[]
  SynInfo : DSPBAPrim/SynthesisInfo  primtype=synthinfo  nInputs=0  nOutputs=0  omode=Inherit via internal rule  otype=sfix(16)  scale=2^-15  rndmethod=Truncate  factor=1  satmethod=Symmetric  shift_vec=[0 1 2 -1]  value=99  inPortNames=[' '; ' ';]  outPortNames=[' ']  dspbaimage=dspba_prim_ctrl.jpg  text=fprintf('Style=%s', style);  style=Scheduled  visibilities=2^17+2^18+2^19+2^20  constraintPair=None  constraintRelation=>  constraintLimit=4  modelRefSign=+  modelRef=''  showSchedule=off  simulationMode=Use Global Value  resetMinimization=Off  version=20220106
  din_a1 : Outport
  vin_a1 : Outport  Port=2
  cin_a1 : Outport  Port=3
  wires:
  Channel_out_HC_Bypass/2 -> cin_a1/1
  Channel_out_HC_Bypass/1 -> vin_a1/1
  Channel_out_HC_Bypass/3 -> din_a1/1
  Channel_In_HB_Bypass/3 -> Mux/2
  SampleDelay/1 -> BitExtract1/1
  din_d1/1 -> Channel_In_HB_Bypass/3
  din_d2/1 -> Channel_In_HB_Bypass/5
  vin_d1/1 -> Channel_In_HB_Bypass/1
  cin_d1/1 -> Channel_In_HB_Bypass/2
  Mux/1 -> Channel_out_HC_Bypass/3
  Channel_In_HB_Bypass/1 -> Channel_out_HC_Bypass/1
  Channel_In_HB_Bypass/2 -> Channel_out_HC_Bypass/2
  RegField/1 -> SampleDelay/1
  mux_sel/1 -> Channel_In_HB_Bypass/4
  Channel_In_HB_Bypass/4 -> Mux/1
  Channel_In_HB_Bypass/5 -> Mux/3

== system ddc_model/DUT/DUT/DDC_l1  ==
  d : Inport
  v : Inport  Port=2
  c : Inport  Port=3
  HB1 : Subsystem
  HB2 : Subsystem
  routing_reg_hb62hb7 : Subsystem
  q : Outport
  qv : Outport  Port=2
  qc : Outport  Port=3
  wires:
  d/1 -> HB2/1(d)
  c/1 -> HB2/2(c)
  HB2/1(q) -> routing_reg_hb62hb7/1(d)
  HB1/1(q) -> q/1
  HB1/2(qv) -> qv/1
  HB1/3(qc) -> qc/1
  routing_reg_hb62hb7/1(q0) -> HB1/1(d)
  HB2/2(qv) -> routing_reg_hb62hb7/2(dv)
  HB2/3(qc) -> routing_reg_hb62hb7/3(dc)
  routing_reg_hb62hb7/2(qv) -> HB1/2(v)
  routing_reg_hb62hb7/3(qc) -> HB1/3(c)
  v/1 -> HB2/3(v)

== system ddc_model/DUT/DUT/enb_subsys1 ==
  In_d : Inport
  Enable : EnablePort
  To Workspace : ToWorkspace  VariableName=polyphase_dec_din  SampleTime=-1
      settings: Save2DSignal=2-D array (concatenate along first dimension)
  wires:
  In_d/1 -> To Workspace/1

== system ddc_model/DUT/DUT/enb_subsys2 ==
  In1 : Inport
  Enable : EnablePort
  To Workspace : ToWorkspace  VariableName=mixer_out1  SampleTime=-1
      settings: Save2DSignal=2-D array (concatenate along first dimension)
  wires:
  In1/1 -> To Workspace/1

== system ddc_model/DUT/DUT/enb_subsys4 ==
  In1 : Inport
  Enable : EnablePort
  To Workspace : ToWorkspace  VariableName=chFiltIn  SampleTime=-1
      settings: Save2DSignal=2-D array (concatenate along first dimension)
  wires:
  In1/1 -> To Workspace/1

== system ddc_model/DUT/DUT/enb_subsys5 ==
  din : Inport
  cin : Inport  Port=2
  Enable : EnablePort
  To Workspace : ToWorkspace  VariableName=chFiltOut  SampleTime=-1
      settings: Save2DSignal=2-D array (concatenate along first dimension)
  To Workspace1 : ToWorkspace  VariableName=chFiltOut_cout  SampleTime=-1
      settings: Save2DSignal=2-D array (concatenate along first dimension)
  wires:
  din/1 -> To Workspace/1
  cin/1 -> To Workspace1/1

== system ddc_model/DUT/DUT/routing_reg_hb72chan_l1 ==
  d : Inport
  dv : Inport  Port=2
  dc : Inport  Port=3
  ChannelIn : DSPBAPrim/ChannelIn  primtype=channelin  nInputs=dspba_internal_get_channel_ports(gcb)  nOutputs=dspba_internal_get_channel_ports(gcb)  omode=Inherit via internal rule  otype=sfix(16)  scale=2^-15  rndmethod=Unbiased  factor=1  satmethod=Symmetric  shift_vec=[0 1 2 -1]  value=1  inPortNames=['v'; 'c'; '0'; '1'; '2'; '3'; '4'; '5'; '6'; '7'; '8'; '9'; 'A'; 'B'; 'D'; 'E'; 'F'; 'G'; 'H'; 'I'; 'J'; 'K'; 'L'; 'M'; 'N'; 'O'; 'P'; 'Q'; 'R'; 'S'; 'T'; 'U'; 'W'; 'X'; 'Y'; 'Z']  outPortNames=['v'; 'c'; '0'; '1'; '2'; '3'; '4'; '5'; '6'; '7'; '8'; '9'; 'A'; 'B'; 'D'; 'E'; 'F'; 'G'; 'H'; 'I'; 'J'; 'K'; 'L'; 'M'; 'N'; 'O'; 'P'; 'Q'; 'R'; 'S'; 'T'; 'U'; 'W'; 'X'; 'Y'; 'Z']  dspbaimage=dspba_prim_channel_tall.svg  text=fprintf('In');  style=Optimised  dataSignals=1  foldingEnabled=off  channels=1  sampleRate=200  packetBeginPresent=off  packetBeginEnabled=off  visibilities=dspba_ChannelInVis(gcb)  scheduleOrigin=on  version=20211214
  ChannelOut : DSPBAPrim/ChannelOut  primtype=channelout  nInputs=dspba_internal_get_channel_ports(gcb)  nOutputs=dspba_internal_get_channel_ports(gcb)  omode=Inherit via internal rule  otype=sfix(16)  scale=2^-15  rndmethod=Unbiased  factor=1  satmethod=Symmetric  shift_vec=[0 1 2 -1]  value=1  inPortNames=['v'; 'c'; '0'; '1'; '2'; '3'; '4'; '5'; '6'; '7'; '8'; '9'; 'A'; 'B'; 'D'; 'E'; 'F'; 'G'; 'H'; 'I'; 'J'; 'K'; 'L'; 'M'; 'N'; 'O'; 'P'; 'Q'; 'R'; 'S'; 'T'; 'U'; 'W'; 'X'; 'Y'; 'Z']  outPortNames=['v'; 'c'; '0'; '1'; '2'; '3'; '4'; '5'; '6'; '7'; '8'; '9'; 'A'; 'B'; 'D'; 'E'; 'F'; 'G'; 'H'; 'I'; 'J'; 'K'; 'L'; 'M'; 'N'; 'O'; 'P'; 'Q'; 'R'; 'S'; 'T'; 'U'; 'W'; 'X'; 'Y'; 'Z']  dspbaimage=dspba_prim_channel_tall.svg  text=fprintf('Out%s', AdvDSPBChannelOutDisplay(latency));  style=Optimised  dataSignals=1  foldingEnabled=off  channels=1  sampleRate=200  packetBeginPresent=off  packetBeginEnabled=off  visibilities=dspba_ChannelOutVis(gcb)  latency=3  version=20211214
  SynthesisInfo : DSPBAPrim/SynthesisInfo  primtype=synthinfo  nInputs=0  nOutputs=0  omode=Inherit via internal rule  otype=sfix(16)  scale=2^-15  rndmethod=Truncate  factor=1  satmethod=Symmetric  shift_vec=[0 1 2 -1]  value=99  inPortNames=[' '; ' ';]  outPortNames=[' ']  dspbaimage=dspba_prim_ctrl.jpg  text=fprintf('Style=%s', style);  style=Scheduled  visibilities=2^17+2^18+2^19+2^20  constraintPair=Channel-In to Channel-Out  constraintRelation=>  constraintLimit=2  modelRefSign=+  modelRef=''  showSchedule=off  simulationMode=Use Global Value  resetMinimization=Conditional - On for ChannelIn/Out only  version=20220106
  q0 : Outport
  qv : Outport  Port=2
  qc : Outport  Port=3
  wires:
  dv/1 -> ChannelIn/1
  d/1 -> ChannelIn/3
  ChannelIn/1 -> ChannelOut/1
  ChannelIn/2 -> ChannelOut/2
  ChannelIn/3 -> ChannelOut/3
  ChannelOut/3 -> q0/1
  ChannelOut/1 -> qv/1
  ChannelOut/2 -> qc/1
  dc/1 -> ChannelIn/2

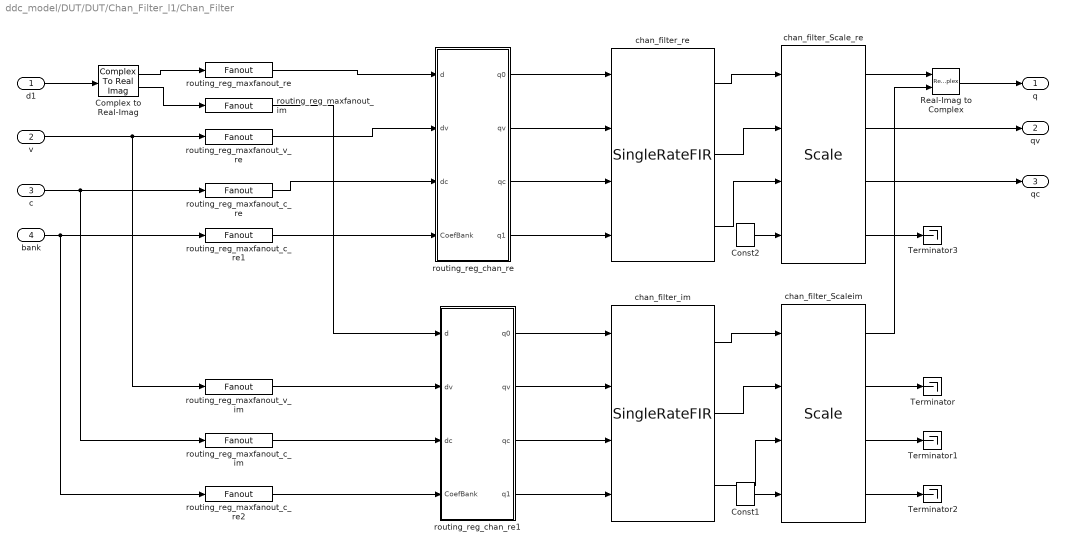
== system ddc_model/DUT/DUT/Chan_Filter_l1/Chan_Filter ==
  d1 : Inport
  v : Inport  Port=2
  c : Inport  Port=3
  bank : Inport  Port=4
  Complex to Real-Imag : ComplexToRealImag
  Const1 : DSPBAPrim/Const  primtype=const  nInputs=0  nOutputs=1  omode=Inherit via internal rule  otype=sfix(16)  scale=2^-15  rndmethod=Unbiased  factor=1  satmethod=Symmetric  shift_vec=[0 1 2 -1]  value=0  inPortNames=['+'; '+';]  outPortNames=[' ']  dspbaimage=dspba_prim.svg  text=fprintf('%s', num2str(value));  style=Optimised  visibilities=8 + 1024  floatPrecision=float32_m23  warnSaturation=on  version=20211007  SampleTime=inf
  Const2 : DSPBAPrim/Const  primtype=const  nInputs=0  nOutputs=1  omode=Inherit via internal rule  otype=sfix(16)  scale=2^-15  rndmethod=Unbiased  factor=1  satmethod=Symmetric  shift_vec=[0 1 2 -1]  value=0  inPortNames=['+'; '+';]  outPortNames=[' ']  dspbaimage=dspba_prim.svg  text=fprintf('%s', num2str(value));  style=Optimised  visibilities=8 + 1024  floatPrecision=float32_m23  warnSaturation=on  version=20211007  SampleTime=inf
  Real-Imag to Complex : RealImagToComplex
  Terminator{,1..3} (4 alike) : Terminator
  chan_filter_Scale_re : DSPBABase/Scale  otype=sfix(output_word_length)  scale=2^-output_fraction_length  rndmethod=Biased  factor=1  satmethod=None  shift_vec=0  latency=2  simulationMode=Use Global Value  version=20130807
  chan_filter_Scaleim : DSPBABase/Scale  otype=sfix(output_word_length)  scale=2^-output_fraction_length  rndmethod=Biased  factor=1  satmethod=None  shift_vec=0  latency=2  simulationMode=Use Global Value  version=20130807
  chan_filter_im : DSPBAFilters/SingleRateFIR  nInputRate=CH_filter_SampleRate  nchan=CH_filter_ChanCount  symmetry=Symmetrical  coef=CH_filter_coeffs  addr=CH_filter_base_addr_l1_im  rwmode=Read/Write  nband=Use All Taps  latency=16  exposebus=off  version=20090407  recon=off  MM=[0,1,2,3,4,5,6,7,8,9,10,11,12,13,14,15,16,17,18,19]  resetrezero=off  sharecoef=auto  simulationMode=Standard
  chan_filter_re : DSPBAFilters/SingleRateFIR  nInputRate=CH_filter_SampleRate  nchan=CH_filter_ChanCount  symmetry=Symmetrical  coef=CH_filter_coeffs  addr=CH_filter_base_addr_l1_re  rwmode=Read/Write  nband=Use All Taps  latency=16  exposebus=off  version=20090407  recon=off  MM=[0,1,2,3,4,5,6,7,8,9,10,11,12,13,14,15,16,17,18,19]  resetrezero=off  sharecoef=auto  simulationMode=Standard
  routing_reg_chan_re : Subsystem
  routing_reg_chan_re1 : Subsystem
  routing_reg_maxfanout_c_im : DSPBAPrim/Fanout  primtype=fanout  nInputs=1  nOutputs=evalAionMaskParam(gcb,'value',1)  omode=Inherit via internal rule  otype=sfix(16)  scale=2^-15  rndmethod=Unbiased  factor=1  satmethod=Symmetric  shift_vec=[0 1 2 -1]  value=1  inPortNames=[' '; ' ';]  outPortNames=[' ']  dspbaimage=dspba_prim_tall.svg  text=fprintf('fanout')  style=Optimised  visibilities=2^10+2^18  version=20211007  uninit=off
  routing_reg_maxfanout_c_re : DSPBAPrim/Fanout  primtype=fanout  nInputs=1  nOutputs=evalAionMaskParam(gcb,'value',1)  omode=Inherit via internal rule  otype=sfix(16)  scale=2^-15  rndmethod=Unbiased  factor=1  satmethod=Symmetric  shift_vec=[0 1 2 -1]  value=1  inPortNames=[' '; ' ';]  outPortNames=[' ']  dspbaimage=dspba_prim_tall.svg  text=fprintf('fanout')  style=Optimised  visibilities=2^10+2^18  version=20211007  uninit=off
  routing_reg_maxfanout_c_re1 : DSPBAPrim/Fanout  primtype=fanout  nInputs=1  nOutputs=evalAionMaskParam(gcb,'value',1)  omode=Inherit via internal rule  otype=sfix(16)  scale=2^-15  rndmethod=Unbiased  factor=1  satmethod=Symmetric  shift_vec=[0 1 2 -1]  value=1  inPortNames=[' '; ' ';]  outPortNames=[' ']  dspbaimage=dspba_prim_tall.svg  text=fprintf('fanout')  style=Optimised  visibilities=2^10+2^18  version=20211007  uninit=off
  routing_reg_maxfanout_c_re2 : DSPBAPrim/Fanout  primtype=fanout  nInputs=1  nOutputs=evalAionMaskParam(gcb,'value',1)  omode=Inherit via internal rule  otype=sfix(16)  scale=2^-15  rndmethod=Unbiased  factor=1  satmethod=Symmetric  shift_vec=[0 1 2 -1]  value=1  inPortNames=[' '; ' ';]  outPortNames=[' ']  dspbaimage=dspba_prim_tall.svg  text=fprintf('fanout')  style=Optimised  visibilities=2^10+2^18  version=20211007  uninit=off
  routing_reg_maxfanout_im : DSPBAPrim/Fanout  primtype=fanout  nInputs=1  nOutputs=evalAionMaskParam(gcb,'value',1)  omode=Inherit via internal rule  otype=sfix(16)  scale=2^-15  rndmethod=Unbiased  factor=1  satmethod=Symmetric  shift_vec=[0 1 2 -1]  value=1  inPortNames=[' '; ' ';]  outPortNames=[' ']  dspbaimage=dspba_prim_tall.svg  text=fprintf('fanout')  style=Optimised  visibilities=2^10+2^18  version=20211007  uninit=off
  routing_reg_maxfanout_re : DSPBAPrim/Fanout  primtype=fanout  nInputs=1  nOutputs=evalAionMaskParam(gcb,'value',1)  omode=Inherit via internal rule  otype=sfix(16)  scale=2^-15  rndmethod=Unbiased  factor=1  satmethod=Symmetric  shift_vec=[0 1 2 -1]  value=1  inPortNames=[' '; ' ';]  outPortNames=[' ']  dspbaimage=dspba_prim_tall.svg  text=fprintf('fanout')  style=Optimised  visibilities=2^10+2^18  version=20211007  uninit=off
  routing_reg_maxfanout_v_im : DSPBAPrim/Fanout  primtype=fanout  nInputs=1  nOutputs=evalAionMaskParam(gcb,'value',1)  omode=Inherit via internal rule  otype=sfix(16)  scale=2^-15  rndmethod=Unbiased  factor=1  satmethod=Symmetric  shift_vec=[0 1 2 -1]  value=1  inPortNames=[' '; ' ';]  outPortNames=[' ']  dspbaimage=dspba_prim_tall.svg  text=fprintf('fanout')  style=Optimised  visibilities=2^10+2^18  version=20211007  uninit=off
  routing_reg_maxfanout_v_re : DSPBAPrim/Fanout  primtype=fanout  nInputs=1  nOutputs=evalAionMaskParam(gcb,'value',1)  omode=Inherit via internal rule  otype=sfix(16)  scale=2^-15  rndmethod=Unbiased  factor=1  satmethod=Symmetric  shift_vec=[0 1 2 -1]  value=1  inPortNames=[' '; ' ';]  outPortNames=[' ']  dspbaimage=dspba_prim_tall.svg  text=fprintf('fanout')  style=Optimised  visibilities=2^10+2^18  version=20211007  uninit=off
  q : Outport
  qv : Outport  Port=2
  qc : Outport  Port=3
  wires:
  chan_filter_re/1 -> chan_filter_Scale_re/1
  Const2/1 -> chan_filter_Scale_re/4
  chan_filter_re/3 -> chan_filter_Scale_re/3
  chan_filter_re/2 -> chan_filter_Scale_re/2
  chan_filter_im/2 -> chan_filter_Scaleim/2
  chan_filter_im/3 -> chan_filter_Scaleim/3
  Const1/1 -> chan_filter_Scaleim/4
  chan_filter_im/1 -> chan_filter_Scaleim/1
  chan_filter_Scaleim/2 -> Terminator/1
  chan_filter_Scaleim/3 -> Terminator1/1
  chan_filter_Scaleim/4 -> Terminator2/1
  chan_filter_Scale_re/4 -> Terminator3/1
  c/1 -> routing_reg_maxfanout_c_im/1, routing_reg_maxfanout_c_re/1
  v/1 -> routing_reg_maxfanout_v_im/1, routing_reg_maxfanout_v_re/1
  Complex to Real-Imag/1 -> routing_reg_maxfanout_re/1
  Complex to Real-Imag/2 -> routing_reg_maxfanout_im/1
  d1/1 -> Complex to Real-Imag/1
  chan_filter_Scale_re/1 -> Real-Imag to Complex/1
  chan_filter_Scaleim/1 -> Real-Imag to Complex/2
  Real-Imag to Complex/1 -> q/1
  chan_filter_Scale_re/3 -> qc/1
  chan_filter_Scale_re/2 -> qv/1
  routing_reg_maxfanout_v_re/1 -> routing_reg_chan_re/2(dv)
  routing_reg_maxfanout_im/1 -> routing_reg_chan_re1/1(d)
  routing_reg_maxfanout_re/1 -> routing_reg_chan_re/1(d)
  routing_reg_maxfanout_c_re/1 -> routing_reg_chan_re/3(dc)
  routing_reg_maxfanout_v_im/1 -> routing_reg_chan_re1/2(dv)
  routing_reg_maxfanout_c_im/1 -> routing_reg_chan_re1/3(dc)
  routing_reg_chan_re/1(q0) -> chan_filter_re/1
  routing_reg_chan_re/2(qv) -> chan_filter_re/2
  routing_reg_chan_re/3(qc) -> chan_filter_re/3
  routing_reg_chan_re1/1(q0) -> chan_filter_im/1
  routing_reg_chan_re1/2(qv) -> chan_filter_im/2
  routing_reg_chan_re1/3(qc) -> chan_filter_im/3
  bank/1 -> routing_reg_maxfanout_c_re2/1, routing_reg_maxfanout_c_re1/1
  routing_reg_maxfanout_c_re1/1 -> routing_reg_chan_re/4(CoefBank)
  routing_reg_maxfanout_c_re2/1 -> routing_reg_chan_re1/4(CoefBank)
  routing_reg_chan_re/4(q1) -> chan_filter_re/4
  routing_reg_chan_re1/4(q1) -> chan_filter_im/4

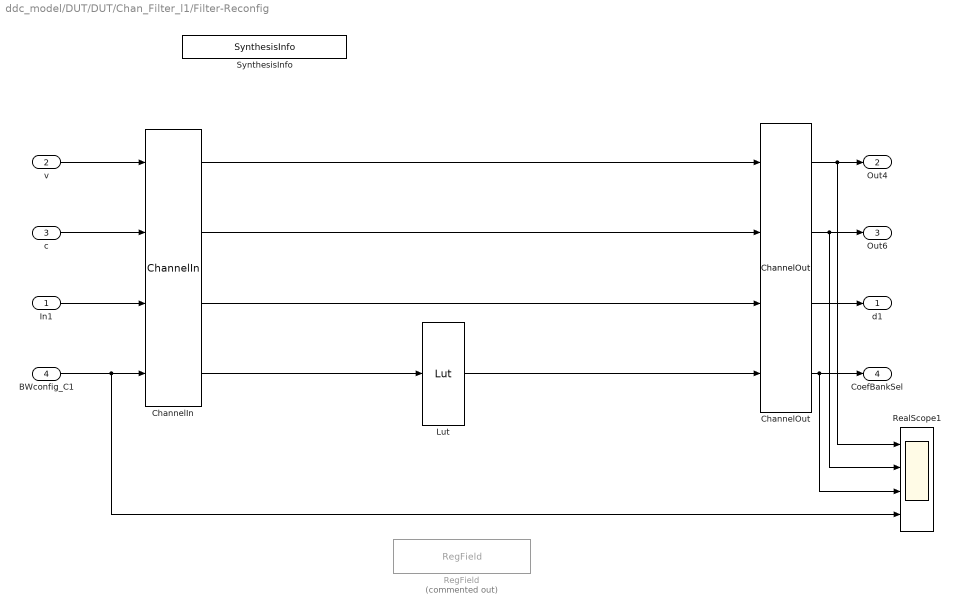
== system ddc_model/DUT/DUT/Chan_Filter_l1/Filter-Reconfig ==
  In1 : Inport
  v : Inport  Port=2
  c : Inport  Port=3
  BWconfig_C1 : Inport  Port=4
  ChannelIn : DSPBAPrim/ChannelIn  primtype=channelin  nInputs=dspba_internal_get_channel_ports(gcb)  nOutputs=dspba_internal_get_channel_ports(gcb)  omode=Inherit via internal rule  otype=sfix(16)  scale=2^-15  rndmethod=Unbiased  factor=1  satmethod=Symmetric  shift_vec=[0 1 2 -1]  value=2  inPortNames=['v'; 'c'; '0'; '1'; '2'; '3'; '4'; '5'; '6'; '7'; '8'; '9'; 'A'; 'B'; 'D'; 'E'; 'F'; 'G'; 'H'; 'I'; 'J'; 'K'; 'L'; 'M'; 'N'; 'O'; 'P'; 'Q'; 'R'; 'S'; 'T'; 'U'; 'W'; 'X'; 'Y'; 'Z']  outPortNames=['v'; 'c'; '0'; '1'; '2'; '3'; '4'; '5'; '6'; '7'; '8'; '9'; 'A'; 'B'; 'D'; 'E'; 'F'; 'G'; 'H'; 'I'; 'J'; 'K'; 'L'; 'M'; 'N'; 'O'; 'P'; 'Q'; 'R'; 'S'; 'T'; 'U'; 'W'; 'X'; 'Y'; 'Z']  dspbaimage=dspba_prim_channel_tall.svg  text=fprintf('In');  style=Optimised  dataSignals=2  foldingEnabled=off  channels=1  sampleRate=200  packetBeginPresent=off  packetBeginEnabled=off  visibilities=dspba_ChannelInVis(gcb)  scheduleOrigin=on  version=20211214
  ChannelOut : DSPBAPrim/ChannelOut  primtype=channelout  nInputs=dspba_internal_get_channel_ports(gcb)  nOutputs=dspba_internal_get_channel_ports(gcb)  omode=Inherit via internal rule  otype=sfix(16)  scale=2^-15  rndmethod=Unbiased  factor=1  satmethod=Symmetric  shift_vec=[0 1 2 -1]  value=2  inPortNames=['v'; 'c'; '0'; '1'; '2'; '3'; '4'; '5'; '6'; '7'; '8'; '9'; 'A'; 'B'; 'D'; 'E'; 'F'; 'G'; 'H'; 'I'; 'J'; 'K'; 'L'; 'M'; 'N'; 'O'; 'P'; 'Q'; 'R'; 'S'; 'T'; 'U'; 'W'; 'X'; 'Y'; 'Z']  outPortNames=['v'; 'c'; '0'; '1'; '2'; '3'; '4'; '5'; '6'; '7'; '8'; '9'; 'A'; 'B'; 'D'; 'E'; 'F'; 'G'; 'H'; 'I'; 'J'; 'K'; 'L'; 'M'; 'N'; 'O'; 'P'; 'Q'; 'R'; 'S'; 'T'; 'U'; 'W'; 'X'; 'Y'; 'Z']  dspbaimage=dspba_prim_channel_tall.svg  text=fprintf('Out%s', AdvDSPBChannelOutDisplay(latency));  style=Optimised  dataSignals=2  foldingEnabled=off  channels=1  sampleRate=200  packetBeginPresent=off  packetBeginEnabled=off  visibilities=dspba_ChannelOutVis(gcb)  latency=2  version=20211214
  Lut : DSPBAPrim/Lut  primtype=lut  nInputs=1  nOutputs=1  omode=Inherit via internal rule  otype=sfix(16)  scale=2^-15  rndmethod=Unbiased  factor=1  satmethod=Symmetric  shift_vec=[0 1 2 -1]  value=[0 0 0 0 0 0 0 0 0 0 0 0 0 0 1 zeros(1,241)]  inPortNames=[' '; ' ';]  outPortNames=[' ']  dspbaimage=dspba_prim.svg  text=fprintf('LUT');  style=Optimised  visibilities=8 + 1024  floatPrecision=float32_m23  version=20211007
  RealScope1 : Scope  NumInputPorts=4
  RegField : DSPBAModelBus/RegField  Commented=on  reg_name=BW_Config_CC1_Offset  reg_rwmode=Read/Write  reg_msb=7  reg_lsb=0  reg_mode=Specify via dialog  reg_type=ufix(8)  reg_scale=2^0  reg_init=BW_Config_CC1  reg_desc=BW Configuration Register for CC1  reg_modal=off  reg_desc0=0  reg_desc1=0  reg_desc2=0  reg_desc3=0  reg_desc4=0  reg_desc5=0  reg_desc6=0  reg_desc7=0  reg_addr=0  SampleTime=-1  version=20090407
  SynthesisInfo : DSPBAPrim/SynthesisInfo  primtype=synthinfo  nInputs=0  nOutputs=0  omode=Inherit via internal rule  otype=sfix(16)  scale=2^-15  rndmethod=Truncate  factor=1  satmethod=Symmetric  shift_vec=[0 1 2 -1]  value=99  inPortNames=[' '; ' ';]  outPortNames=[' ']  dspbaimage=dspba_prim_ctrl.jpg  text=fprintf('Style=%s', style);  style=Scheduled  visibilities=2^15+2^17+2^18+2^19  constraintPair=None  constraintRelation=>  constraintLimit=Latency  modelRefSign=+  modelRef=''  showSchedule=off  simulationMode=Use Global Value  resetMinimization=Conditional - On for ChannelIn/Out only  version=20220106
  d1 : Outport
  Out4 : Outport  Port=2
  Out6 : Outport  Port=3
  CoefBankSel : Outport  Port=4
  wires:
  ChannelOut/2 -> RealScope1/2, Out6/1
  v/1 -> ChannelIn/1
  In1/1 -> ChannelIn/3
  c/1 -> ChannelIn/2
  ChannelOut/1 -> RealScope1/1, Out4/1
  ChannelOut/3 -> d1/1
  ChannelOut/4 -> RealScope1/3, CoefBankSel/1
  ChannelIn/4 -> Lut/1
  Lut/1 -> ChannelOut/4
  ChannelIn/1 -> ChannelOut/1
  ChannelIn/2 -> ChannelOut/2
  ChannelIn/3 -> ChannelOut/3
  BWconfig_C1/1 -> RealScope1/4, ChannelIn/4
